simulink model "ADT_SimulinkModel"  (R2023b)
settings: Solver=VariableStepAuto  StartTime=0.0  StopTime=150  RelTol=1e-3
values from neighbouring files (symbols this model uses):
  cx = 640    [variablesInitialization.m]
  cy = 360    [variablesInitialization.m]
  fx = 1109    [variablesInitialization.m]
  fy = 1109    [variablesInitialization.m]
  refX = UsCityBlockPose(:,1)    [variablesInitialization.m]
  refY = UsCityBlockPose(:,2)    [variablesInitialization.m]
  refYaw = UsCityBlockPose(:,3)    [variablesInitialization.m]
  Ts = timeVector(3) - timeVector(2)    [variablesInitialization.m]
undefined symbols (not defined in the file or in its folder): DiscIntNeverNeededParam, fractalcoef
libraries: simulink x3, sim3dcameralib x1, sensorgpslib x1, mspsensorlib x1, sensorinslib x1, sim3dphyssensorlib x1, sim3dlib x1, sim3dautolib x1, dspvision x1
settings Model: Creator=YOUSRA  LastModifiedBy=Hazem Abdelaziz

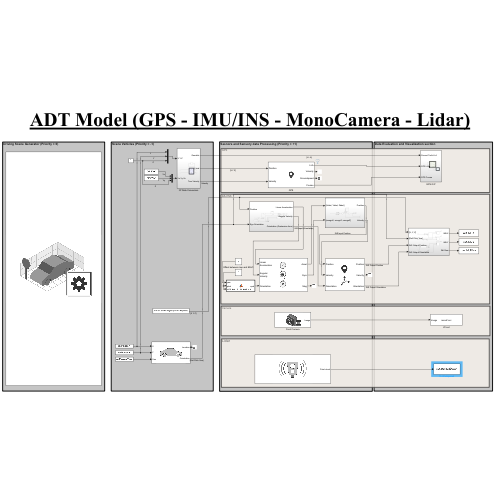
[thumbnail: Simulink's stored preview of the top-level diagram]
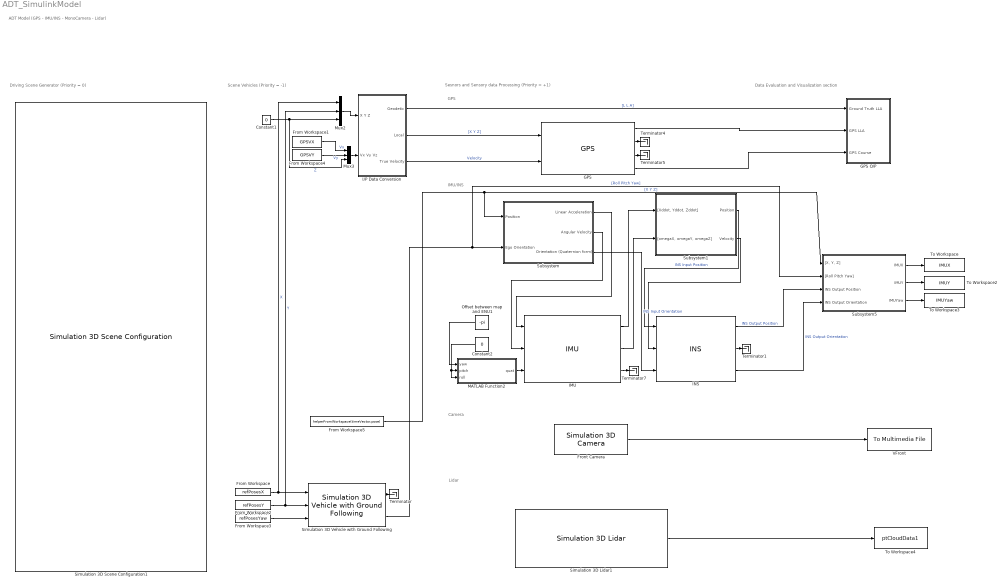
== system ADT_SimulinkModel ==
  note: GPS
  note: IMU/INS
  note: Camera
  note: Driving Scene Generator (Priority = 0)
  note: Scene Vehicles (Priority = -1)
  note: Data Evaluation and Visualization section
  note: Sesnors and Sensory data Processing (Priority = +1)
  note: ADT Model (GPS - IMU/INS - MonoCamera - Lidar)
  note: Lidar
  Constant1 : Constant  Value=0
  Constant2 : Constant  Priority=1  Value=0
  From Workspace : FromWorkspace  VariableName=refPosesX  SampleTime=Ts
  From Workspace1 : FromWorkspace  VariableName=GPSVX  SampleTime=Ts
  From Workspace2 : FromWorkspace  VariableName=refPosesY  SampleTime=Ts
  From Workspace3 : FromWorkspace  VariableName=refPosesYaw  SampleTime=Ts
  From Workspace4 : FromWorkspace  VariableName=GPSVY  SampleTime=Ts
  From Workspace5 : FromWorkspace  VariableName=helperFromWorkspace(timeVector,pose)  SampleTime=Ts
  Front Camera : sim3dcameralib/Simulation 3D Camera  Priority=1  sensorTag=Sim3dSensor2  sensorId=2  sensorName=Sim3dSensor2  vehTagList={'Scene Origin';'SimulinkVehicle2'}  vehTag=SimulinkVehicle2  mountLoc=Roof center  offsetFlag=off  tmountOffset=[0, 0.06, 0]  extTmount=off  rmountOffset=[0, 0, -0.2611]  extRmount=off  FocalLength=[fx, fy]  OpticalCenter=[cx, cy]  ImageSize=[720 1280]  RadialDistortion=[0, 0]  TangentialDistortion=[0, 0]  SensorSkew=0  DepthOutportEnabled=off  SemanticOutportEnabled=off  TransformOutportEnabled=off  SampleTime=-1  mountPoint=[-0.560000002384186 0 1.99000000953674]  mountOrientation=[0 0 0]  aMode=3  ID=2
      settings: LibrarySourceBlock=drivingsim3d/Simulation 3D Camera
  GPS : sensorgpslib/GPS  DispRefFrame=NED  PositionInputFormat=Local  ReferenceLocation=[ 0, 0, 0]  HorizontalPositionAccuracy=0.1  VerticalPositionAccuracy=0.1  VelocityAccuracy=0.01  DecayFactor=0.999  SeedDouble=0  SimulateUsing=Interpreted execution
  GPS O/P : Subsystem
  I/P Data Conversion : Subsystem
  IMU : mspsensorlib/IMU  Priority=1  DispRefFrame=ENU  TemperaturePort=off  Temperature=25  MagneticFieldPort=off  MagneticFieldNED=[ 27.5550, -2.4169, -16.0849 ]  MagneticFieldENU=[-2.4169, 27.5550, 16.0849]  SeedDouble=0  SimulateUsing=Interpreted execution  AccelParamsMeasurementRange=Inf  AccelParamsResolution=0  AccelParamsConstantBias=[ 0, 0, 9.80 ]  AccelParamsAxesMisalignment=[ 100, 0, 0; 0, 100, 0; 0, 0, 100 ]  AccelParamsNoiseDensity=[ 0, 0, 0 ]  AccelParamsBiasInstability=[ 0, 0, 0 ]  AccelParamsBiasInstabilityNumerator=fractalcoef().Numerator  AccelParamsBiasInstabilityDenominator=fractalcoef().Denominator  AccelParamsRandomWalk=[ 0, 0, 0 ]  AccelParamsNoiseType=double-sided  AccelParamsTemperatureBias=[ 0, 0, 0 ]  AccelParamsTemperatureScaleFactor=[ 0, 0, 0 ]  GyroParamsMeasurementRange=Inf  GyroParamsResolution=0  GyroParamsConstantBias=[ 0, 0, 0 ]  GyroParamsAxesMisalignment=[ 100, 0, 0; 0, 100, 0; 0, 0, 100 ]  GyroParamsAccelerationBias=[ 0, 0, 0 ]  GyroParamsNoiseDensity=[ 0, 0, 0 ]  GyroParamsBiasInstability=[ 0, 0, 0 ]  GyroParamsBiasInstabilityNumerator=fractalcoef().Numerator  GyroParamsBiasInstabilityDenominator=fractalcoef().Denominator  GyroParamsRandomWalk=[ 0, 0, 0 ]  GyroParamsNoiseType=double-sided  GyroParamsTemperatureBias=[ 0, 0, 0 ]  GyroParamsTemperatureScaleFactor=[ 0, 0, 0 ]  MagParamsMeasurementRange=Inf  MagParamsResolution=0  MagParamsConstantBias=[ 0, 0, 0 ]  MagParamsAxesMisalignment=[ 100, 0, 0; 0, 100, 0; 0, 0, 100 ]  MagParamsNoiseDensity=[ 0, 0, 0 ]  MagParamsBiasInstability=[ 0, 0, 0 ]  MagParamsBiasInstabilityNumerator=fractalcoef().Numerator  MagParamsBiasInstabilityDenominator=fractalcoef().Denominator  MagParamsRandomWalk=[ 0, 0, 0 ]  MagParamsNoiseType=double-sided  MagParamsTemperatureBias=[ 0, 0, 0 ]  MagParamsTemperatureScaleFactor=[ 0, 0, 0 ]
  INS : sensorinslib/INS  Priority=1  MountingLocation=[0 0 0]  RollAccuracy=0.05  PitchAccuracy=0.05  YawAccuracy=0.05  PositionAccuracy=0.1  VelocityAccuracy=0.01  UseAccelAndAngVel=off  AccelerationAccuracy=0.1  AngularVelocityAccuracy=0.1  TimeInput=off  PositionErrorFactor=[0 0 0]  SeedDouble=0  SimulateUsing=Interpreted execution
      settings: LibrarySourceBlock=mspsensorlib/INS
  MATLAB Function2 : MATLAB Function  Priority=1  TreatAsAtomicUnit=on
  Mux2 : Mux  Inputs=3
  Mux3 : Mux  Inputs=3
  Offset between map and ENU1 : Constant  Priority=1  Value=-pi
  Simulation 3D Lidar1 : sim3dphyssensorlib/Simulation 3D Lidar  Priority=1  sensorTag=Sim3dSensor4  sensorId=4  sensorName=Sim3dSensor4  vehTagList={'Scene Origin';'SimulinkVehicle2'}  vehTag=SimulinkVehicle2  mountLoc=Roof center  offsetFlag=off  tmountOffset=[0, 0, 0]  rmountOffset=[0, 0, 0]  DetectionRange=120  RangeResolution=0.001  VerticalFOV=Vfov  VerticalResolution=Vres  HorizontalFOV=Hfov  HorizontalResolution=Hres  DistanceOutportEnabled=off  ReflectivityOutportEnabled=off  SemanticOutportEnabled=off  TransformOutportEnabled=off  SampleTime=-1  mountPoint=[-0.560000002384186 0 1.99000000953674]  mountOrientation=[0 0 0]  aMode=3  ID=4
      settings: LibrarySourceBlock=drivingsim3d/Simulation 3D Lidar
  Simulation 3D Scene Configuration1 : sim3dlib/Simulation 3D Scene Configuration  Priority=0  ProjectFormat=Default Scenes  SceneDesc=US city block  ProjectName=C:\Program Files\MATLAB\R2023b\toolbox\shared\sim3d_projects\automotive_project_windows\UE\WindowsNoEditor\VehicleSimulation.exe  ScenePath=/Game/Maps/HwStrght  EnableOpenDRIVE=off  vehTagList={'Custom';'Scene Origin';'SimulinkVehicle2'}  vehTag=SimulinkVehicle2  FreeCameraInitialTranslation=[0, 0, 0]  FreeCameraDefaultInitialTranslation=[-6, 0, 2]  FreeCameraInitialRotation=[0, 0, 0]  FreeCameraDefaultInitialRotation=[0, -15, 0]  OpVisEn=off  Ts=Ts  EnableWindow=on  EnableRemoteAccess=off  EnableWeather=off  SunAltitude=40  SunAzimuth=90  clouds=10  wind=1  fog=0  rain=0  EnableGeospatial=off  OriginHeight=200  OriginLatitude=40.744652  OriginLongitude=-73.988864  MapStyle=Aerial  AdditionalAssetIDs=[]  UseAdvancedSunSky=off  SolarTime=11  TimeZone=-5  Day=21  Month=9  Year=2022  UseDaylightSavingTime=on  DSTStartDay=10  DSTStartMonth=3  DSTEndDay=3  DSTEndMonth=11  DSTSwitchHour=2  sensorTag=MainCamera2  sensorId=2  sensorName=MainCamera2  mountLoc=Origin  offsetFlag=off  tmountOffset=[0, 0, 0]  rmountOffset=[0, 0, 0]  HorizontalResolution=1280  VerticalResolution=720  HorizontalFOV=60  mountPoint=[0 0 0]  mountOrientation=[0 0 0]  aMode=3  ID=2  GeoTrigger=Inactive
      settings: LibrarySourceBlock=drivingsim3d/Simulation 3D Scene Configuration
  Simulation 3D Vehicle with Ground Following : sim3dautolib/Simulation 3D Vehicle with Ground Following  Priority=-1  PassVehMesh=Sport utility vehicle  MeshPath=/MathWorksAutomotiveContent/Vehicles/Muscle/Meshes/SK_MuscleCar.SK_MuscleCar  TrackWidth=1.9  WheelBase=3  WheelRadius=0.35  VehColor=Orange  InitialPos=[refX(1), refY(1), 0]  InitialRot=[0, 0, refYaw(1)]  ActorName=SimulinkVehicle2  SampleTime=-1  ActorType=SimulinkVehicle  ID=2  aMode=3  ActorTag=SimulinkVehicle2  CoordinateScheme=ISO  VehLightsControl=off  HeadlightColor=[ 1, 1, 1 ]  HighBeamIntensity=100000  LowBeamIntensity=60000  HighBeamConeAngle=70  LowBeamConeAngle=70  LeftHeadlightOrientation=[ 0, 0 ]  RightHeadlightOrientation=[ 0, 0 ]  BrakelightIntensity=500  ReverselightIntensity=500  SignallightIntensity=500  SignallightPeriod=1  SignalPulseWidth=50  TransformOutportEnabled=on
      settings: LibrarySourceBlock=drivingsim3d/Simulation 3D Vehicle with Ground Following
  Subsystem : Subsystem  Priority=1
  Subsystem1 : Subsystem  Priority=1
  Subsystem5 : Subsystem
  Terminator{,1,4..5,7} (5 alike) : Terminator
  To Workspace : ToWorkspace  VariableName=IMUX  SaveFormat=Timeseries  SampleTime=-1
  To Workspace2 : ToWorkspace  VariableName=IMUY  SaveFormat=Timeseries  SampleTime=-1
  To Workspace3 : ToWorkspace  VariableName=IMUYaw  SaveFormat=Timeseries  SampleTime=-1
  To Workspace4 : ToWorkspace  VariableName=ptCloudData1  SaveFormat=Structure With Time  SampleTime=-1
  VFront : dspvision/To Multimedia File  outputFilename=CamVideos\monoF.avi  streamSelection=Video only  videoCompressor=None (uncompressed)  audioCompressor=None (uncompressed)  imagePorts=One multidimensional signal  fileType=AVI  audioDatatype=Determine from input data type  fourcc=RGB  videoQuality=75  mj2000CompFactor=10
      settings: LibrarySourceBlock=visionsinks/To Multimedia File
  wires:
  GPS/1 -> GPS O/P/2(GPS LLA)
  GPS/4 -> GPS O/P/3("GPS Course ")
  Front Camera/1 -> VFront/1
  Constant1/1 -> Mux2/3, Mux3/3  "Z"
  Mux2/1 -> I/P Data Conversion/1(X Y Z)
  Mux3/1 -> I/P Data Conversion/2(Vx Vy Vz)
  I/P Data Conversion/1(Geodetic) -> GPS O/P/1(Ground Truth LLA)  "[L L A]"
  I/P Data Conversion/2(Local) -> GPS/1  "[X Y Z]"
  From Workspace2/1 -> Simulation 3D Vehicle with Ground Following/2, Mux2/2  "Y"
  From Workspace3/1 -> Simulation 3D Vehicle with Ground Following/3
  From Workspace/1 -> Mux2/1, Simulation 3D Vehicle with Ground Following/1  "X"
  I/P Data Conversion/3(True Velocity) -> GPS/2  "Velocity"
  From Workspace1/1 -> Mux3/1  "Vx"
  From Workspace4/1 -> Mux3/2  "Vy"
  Simulation 3D Vehicle with Ground Following/1 -> Terminator/1
  Subsystem5/1(IMUX) -> To Workspace/1
  Subsystem5/2(IMUY) -> To Workspace2/1
  Subsystem5/3(IMUYaw) -> To Workspace3/1
  GPS/2 -> Terminator4/1
  GPS/3 -> Terminator5/1
  IMU/2 -> Subsystem1/2("[omegaX, omegaY, omegaZ]")
  IMU/3 -> Terminator7/1
  Subsystem1/2(Velocity) -> INS/2
  Offset between map and ENU1/1 -> MATLAB Function2/1(yaw)
  Subsystem/3(Orientation (Quaternion form)) -> INS/3  "INS Input Orientation"
  Subsystem/2(Angular Velocity) -> IMU/2
  MATLAB Function2/1(quat) -> IMU/3
  Subsystem/1(Linear Acceleration) -> IMU/1
  IMU/1 -> Subsystem1/1("[Xddot, Yddot, Zddot]")
  Subsystem1/1(Position) -> INS/1  "INS Input Position"
  Constant2/1 -> MATLAB Function2/2(pitch), MATLAB Function2/3(roll)
  From Workspace5/1 -> Subsystem/1(Position), Subsystem5/1("[X, Y, Z]")  "[X Y Z]"
  Simulation 3D Vehicle with Ground Following/2 -> Subsystem5/2("[Roll Pitch Yaw]"), Subsystem/2(Ego Orientation)  "[Roll Pitch Yaw]"
  INS/1 -> Subsystem5/3(INS Output Position)  "INS Output Position"
  INS/3 -> Subsystem5/4(INS Output Orientation)  "INS Output Orientation"
  INS/2 -> Terminator1/1
  Simulation 3D Lidar1/1 -> To Workspace4/1

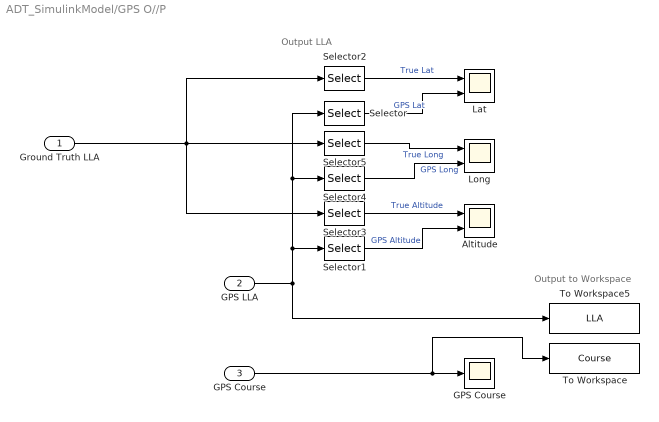
== system ADT_SimulinkModel/GPS O//P ==
  note: Output to Workspace
  note: Output LLA
  Ground Truth LLA : Inport
  GPS LLA : Inport  Port=2
  "GPS Course " : Inport  Port=3
  Altitude : Scope  NumInputPorts=2
  GPS Course : Scope
  Lat : Scope  NumInputPorts=2
  Long : Scope  NumInputPorts=2
  Selector : Selector  InputPortWidth=3  IndexOptions=Index vector (dialog)  Indices=[1]  OutputSizes=1
  Selector1 : Selector  InputPortWidth=3  IndexOptions=Index vector (dialog)  Indices=[3]  OutputSizes=1
  Selector2 : Selector  InputPortWidth=3  IndexOptions=Index vector (dialog)  Indices=[1]  OutputSizes=1
  Selector3 : Selector  InputPortWidth=3  IndexOptions=Index vector (dialog)  Indices=[3]  OutputSizes=1
  Selector4 : Selector  InputPortWidth=3  IndexOptions=Index vector (dialog)  Indices=[2]  OutputSizes=1
  Selector5 : Selector  InputPortWidth=3  IndexOptions=Index vector (dialog)  Indices=[2]  OutputSizes=1
  To Workspace : ToWorkspace  VariableName=Course  SaveFormat=Timeseries  SampleTime=-1
  To Workspace5 : ToWorkspace  VariableName=LLA  SaveFormat=Timeseries  SampleTime=-1
  wires:
  Selector/1 -> Lat/2  "GPS Lat"
  Selector1/1 -> Altitude/2  "GPS Altitude"
  Selector3/1 -> Altitude/1  "True Altitude"
  Ground Truth LLA/1 -> Selector3/1, Selector5/1, Selector2/1
  GPS LLA/1 -> Selector1/1, Selector/1, Selector4/1, To Workspace5/1
  Selector2/1 -> Lat/1  "True Lat"
  "GPS Course "/1 -> To Workspace/1, GPS Course/1
  Selector5/1 -> Long/1  "True Long"
  Selector4/1 -> Long/2  "GPS Long"

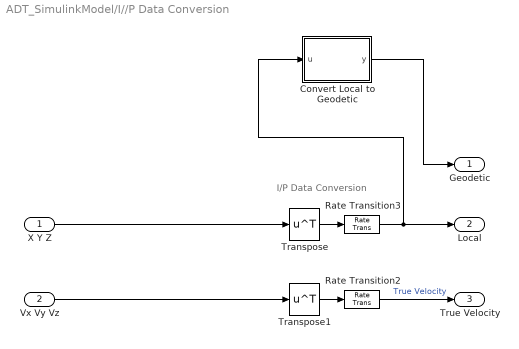
== system ADT_SimulinkModel/I//P Data Conversion ==
  note: I/P Data Conversion
  X Y Z : Inport
  Vx Vy Vz : Inport  Port=2
  Convert Local to Geodetic : MATLAB Function  TreatAsAtomicUnit=on
  Rate Transition2 : RateTransition  OutPortSampleTime=0.1
  Rate Transition3 : RateTransition  OutPortSampleTime=0.1
  Transpose : Math  Operator=transpose
  Transpose1 : Math  Operator=transpose
  Geodetic : Outport
  Local : Outport  Port=2
  True Velocity : Outport  Port=3
  wires:
  Rate Transition3/1 -> Convert Local to Geodetic/1(u), Local/1
  Convert Local to Geodetic/1(y) -> Geodetic/1
  Vx Vy Vz/1 -> Transpose1/1
  Rate Transition2/1 -> True Velocity/1  "True Velocity"
  Transpose/1 -> Rate Transition3/1
  Transpose1/1 -> Rate Transition2/1
  X Y Z/1 -> Transpose/1

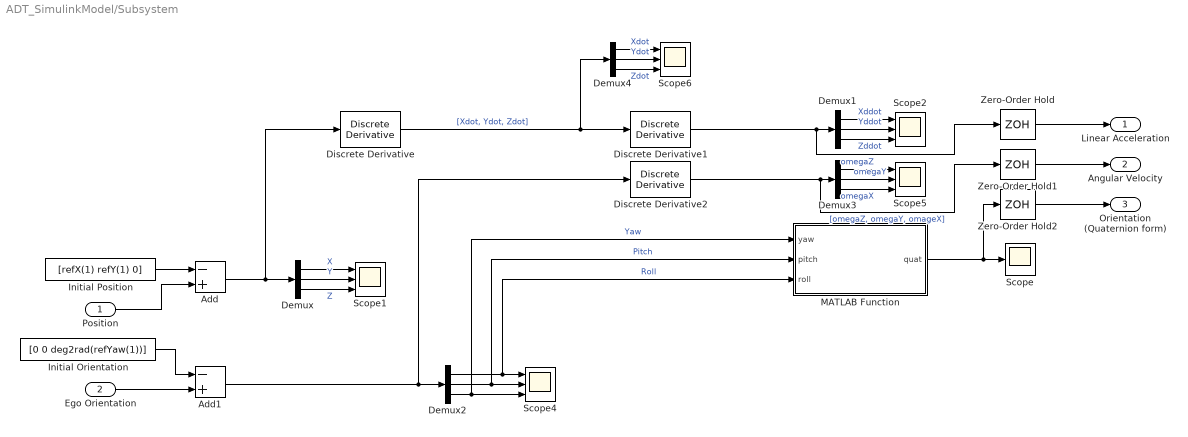
== system ADT_SimulinkModel/Subsystem ==
  Position : Inport
  Ego Orientation : Inport  Port=2
  Add : Sum  Inputs=-+
  Add1 : Sum  Inputs=-+
  Demux{,1..4} (5 alike) : Demux  Outputs=3
  Discrete Derivative : simulink/Discrete/Discrete Derivative  gainval=1.0  ICPrevScaledInput=0  OutMin=[]  OutMax=[]  OutDataType=fixdt(1, 16)  OutScaling=2^-10  DoSatur=off
  Discrete Derivative1 : simulink/Discrete/Discrete Derivative  gainval=1.0  ICPrevScaledInput=0  OutMin=[]  OutMax=[]  OutDataType=fixdt(1, 16)  OutScaling=2^-10  DoSatur=off
  Discrete Derivative2 : simulink/Discrete/Discrete Derivative  gainval=1  ICPrevScaledInput=0  OutMin=[]  OutMax=[]  OutDataType=fixdt(1, 16)  OutScaling=2^-10  DoSatur=off
  Initial Orientation : Constant  Value=[0 0 deg2rad(refYaw(1))]  SampleTime=Ts
  Initial Position : Constant  Value=[refX(1) refY(1) 0]  SampleTime=Ts
  MATLAB Function : MATLAB Function  TreatAsAtomicUnit=on
  Scope : Scope
  Scope{1..2,4..6} (5 alike) : Scope  NumInputPorts=3
  Zero-Order Hold : ZeroOrderHold  SampleTime=Ts
  Zero-Order Hold1 : ZeroOrderHold  SampleTime=Ts
  Zero-Order Hold2 : ZeroOrderHold  SampleTime=Ts
  Linear Acceleration : Outport
  Angular Velocity : Outport  Port=2
  Orientation (Quaternion form) : Outport  Port=3
  wires:
  Demux1/1 -> Scope2/1  "Xddot"
  Demux2/1 -> MATLAB Function/3(roll), Scope4/1  "Roll"
  Discrete Derivative2/1 -> Zero-Order Hold1/1, Demux3/1  "[omegaZ, omegaY, omageX]"
  Demux2/3 -> MATLAB Function/1(yaw), Scope4/3  "Yaw"
  Demux1/3 -> Scope2/3  "Zddot"
  Demux2/2 -> MATLAB Function/2(pitch), Scope4/2  "Pitch"
  Discrete Derivative1/1 -> Zero-Order Hold/1, Demux1/1
  Demux3/3 -> Scope5/3  "omegaX"
  Demux/2 -> Scope1/2  "Y"
  Demux3/1 -> Scope5/1  "omegaZ"
  MATLAB Function/1(quat) -> Zero-Order Hold2/1, Scope/1
  Demux/1 -> Scope1/1  "X"
  Demux1/2 -> Scope2/2  "Yddot"
  Demux3/2 -> Scope5/2  "omegaY"
  Demux/3 -> Scope1/3  "Z"
  Initial Position/1 -> Add/1
  Demux4/1 -> Scope6/1  "Xdot"
  Demux4/2 -> Scope6/2  "Ydot"
  Demux4/3 -> Scope6/3  "Zdot"
  Discrete Derivative/1 -> Demux4/1, Discrete Derivative1/1  "[Xdot, Ydot, Zdot]"
  Zero-Order Hold/1 -> Linear Acceleration/1
  Zero-Order Hold1/1 -> Angular Velocity/1
  Zero-Order Hold2/1 -> Orientation (Quaternion form)/1
  Add/1 -> Discrete Derivative/1, Demux/1
  Position/1 -> Add/2
  Ego Orientation/1 -> Add1/2
  Add1/1 -> Discrete Derivative2/1, Demux2/1
  Initial Orientation/1 -> Add1/1

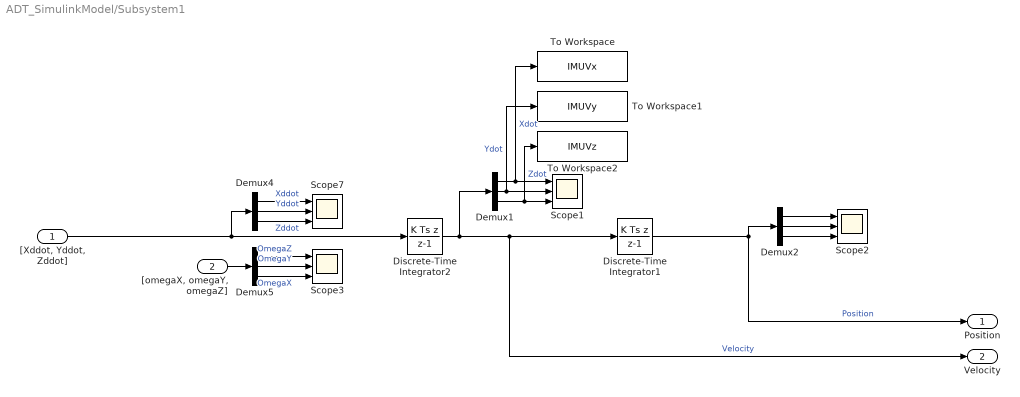
== system ADT_SimulinkModel/Subsystem1 ==
  "[Xddot, Yddot, Zddot]" : Inport
  "[omegaX, omegaY, omegaZ]" : Inport  Port=2
  Demux{1..2,4..5} (4 alike) : Demux  Outputs=3
  Discrete-Time Integrator1 : DiscreteIntegrator  Priority=-1  IntegratorMethod=Integration: Backward Euler  SampleTime=-1  RndMeth=Round  ICPrevOutput=DiscIntNeverNeededParam  ICPrevScaledInput=DiscIntNeverNeededParam
  Discrete-Time Integrator2 : DiscreteIntegrator  Priority=-1  IntegratorMethod=Integration: Backward Euler  SampleTime=-1  ICPrevOutput=DiscIntNeverNeededParam  ICPrevScaledInput=DiscIntNeverNeededParam
  Scope{1..3,7} (4 alike) : Scope  NumInputPorts=3
  To Workspace : ToWorkspace  VariableName=IMUVx  SaveFormat=Timeseries  SampleTime=-1
  To Workspace1 : ToWorkspace  VariableName=IMUVy  SaveFormat=Timeseries  SampleTime=-1
  To Workspace2 : ToWorkspace  VariableName=IMUVz  SaveFormat=Timeseries  SampleTime=-1
  Position : Outport
  Velocity : Outport  Port=2
  wires:
  Demux5/1 -> Scope3/1  "OmegaZ"
  Demux4/2 -> Scope7/2  "Yddot"
  Discrete-Time Integrator2/1 -> Velocity/1, Discrete-Time Integrator1/1, Demux1/1  "Velocity"
  Demux2/3 -> Scope2/3
  Demux4/3 -> Scope7/3  "Zddot"
  Demux5/3 -> Scope3/3  "OmegaX"
  Demux4/1 -> Scope7/1  "Xddot"
  Demux5/2 -> Scope3/2  "OmegaY"
  "[Xddot, Yddot, Zddot]"/1 -> Discrete-Time Integrator2/1, Demux4/1
  Demux2/1 -> Scope2/1
  Demux2/2 -> Scope2/2
  "[omegaX, omegaY, omegaZ]"/1 -> Demux5/1
  Demux1/3 -> Scope1/3, To Workspace2/1  "Zdot"
  Demux1/1 -> Scope1/1, To Workspace/1  "Xdot"
  Demux1/2 -> Scope1/2, To Workspace1/1  "Ydot"
  Discrete-Time Integrator1/1 -> Position/1, Demux2/1  "Position"

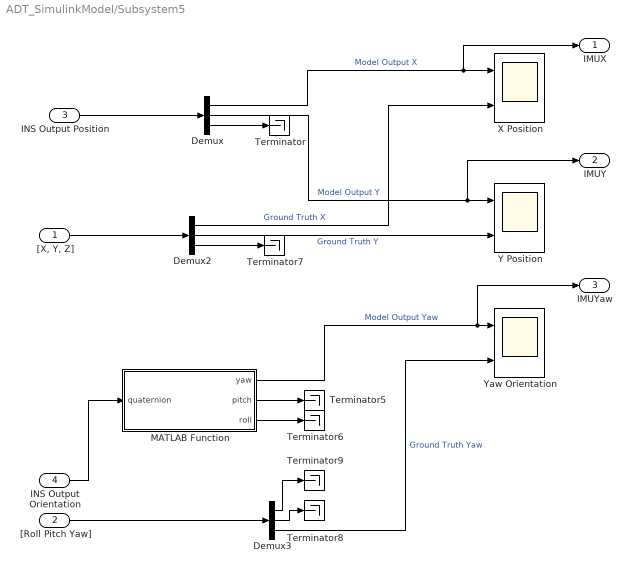
== system ADT_SimulinkModel/Subsystem5 ==
  "[X, Y, Z]" : Inport
  "[Roll Pitch Yaw]" : Inport  Port=2
  INS Output Position : Inport  Port=3
  INS Output Orientation : Inport  Port=4
  Demux : Demux  Outputs=3
  Demux2 : Demux  Outputs=3
  Demux3 : Demux  Outputs=3
  MATLAB Function : MATLAB Function  TreatAsAtomicUnit=on
  Terminator{,5..9} (6 alike) : Terminator
  X Position : Scope  NumInputPorts=2
  Y Position : Scope  NumInputPorts=2
  Yaw Orientation : Scope  NumInputPorts=2
  IMUX : Outport
  IMUY : Outport  Port=2
  IMUYaw : Outport  Port=3
  wires:
  MATLAB Function/1(yaw) -> IMUYaw/1, Yaw Orientation/1  "Model Output Yaw"
  Demux3/2 -> Terminator8/1
  Demux3/3 -> Yaw Orientation/2  "Ground Truth Yaw"
  Demux/1 -> IMUX/1, X Position/1  "Model Output X"
  Demux2/1 -> X Position/2  "Ground Truth X"
  INS Output Orientation/1 -> MATLAB Function/1(quaternion)
  MATLAB Function/2(pitch) -> Terminator5/1
  Demux/2 -> IMUY/1, Y Position/1  "Model Output Y"
  Demux2/2 -> Y Position/2  "Ground Truth Y"
  MATLAB Function/3(roll) -> Terminator6/1
  Demux2/3 -> Terminator7/1
  INS Output Position/1 -> Demux/1
  Demux/3 -> Terminator/1
  Demux3/1 -> Terminator9/1
  "[X, Y, Z]"/1 -> Demux2/1
  "[Roll Pitch Yaw]"/1 -> Demux3/1

== matlab function ADT_SimulinkModel/Subsystem/MATLAB Function ==
  data: yaw input; quat output; pitch input; roll input
function quat = euler_to_quaternion(yaw, pitch, roll)
    %Converting Euler angles to quaternion


    % Compute quaternion components
    cy = cos(yaw * 0.5);
    sy = sin(yaw * 0.5);
    cp = cos(pitch * 0.5);
    sp = sin(pitch * 0.5);
    cr = cos(roll * 0.5);
    sr = sin(roll * 0.5);

    % Quaternion elements
    qw = cy * cp * cr + sy * sp * sr;
    qx = cy * cp * sr - sy * sp * cr;
    qy = sy * cp * sr + cy * sp * cr;
    qz = sy * cp * cr - cy * sp * sr;

    % Output quaternion
    quat = [qw, qx, qy, qz];

== matlab function ADT_SimulinkModel/I//P Data Conversion/Convert Local to Geodetic ==
  data: u input; y output
function y = local2geo(u)

y = ned2lla(u,[0 0 0],"ellipsoid");

end

== matlab function ADT_SimulinkModel/MATLAB Function2 ==
  data: yaw input; quat output; pitch input; roll input
function quat = euler_to_quaternion(yaw, pitch, roll)
    %Converting Euler angles to quaternion


    % Compute quaternion components
    cy = cos(yaw * 0.5);
    sy = sin(yaw * 0.5);
    cp = cos(pitch * 0.5);
    sp = sin(pitch * 0.5);
    cr = cos(roll * 0.5);
    sr = sin(roll * 0.5);

    % Quaternion elements
    qw = cy * cp * cr + sy * sp * sr;
    qx = cy * cp * sr - sy * sp * cr;
    qy = sy * cp * sr + cy * sp * cr;
    qz = sy * cp * cr - cy * sp * sr;

    % Output quaternion
    quat = [qw, qx, qy, qz];

== matlab function ADT_SimulinkModel/Subsystem5/MATLAB Function ==
  data: quaternion input; yaw output; pitch output; roll output
function [yaw, pitch ,roll] = quaternion_to_euler(quaternion)
%Converting quaternion vector to euler angles


    %Extract quaternion components
    q0 = quaternion(1);
    q1 = quaternion(2);
    q2 = quaternion(3);
    q3 = quaternion(4);

    %Euler angles
    yaw = (atan2(2*(q0*q3 + q1*q2), 1 - 2*(q2^2 + q3^2)));
    pitch = asin(2*(q0*q2 - q3*q1));
    roll = atan2(2*(q0*q1 + q2*q3), 1 - 2*(q1^2 + q2^2));
